simulink model "nxtway_gs_plant"  (Simulink 10.0)
settings: Solver=ode45  StartTime=0.0  StopTime=10.0  MaxStep=TS  RelTol=1e-3  EnableMultiTasking=on
PreLoadFcn:
  | param_nxtway_gs
undefined symbols (not defined in the file): A1, A2, B1, B2, C1, C2, D1, D2, X1IV, X2IV
settings Model: Creator=y_yama  LastModifiedBy=bhisma
settings DataIOCC: LimitDataPoints=on  SignalLoggingSaveFormat=ModelDataLogs  SaveOutput=off  SignalLogging=off  SaveTime=off
settings OptimizationCC: DefaultParameterBehavior=Inlined  InlineInvariantSignals=on  ExpressionDepthLimit=2147483647  InitFltsAndDblsToZero=on  LifeSpan=1
settings DebuggingCC: SolverPrmCheckMsg=warning  FcnCallInpInsideContextMsg=warning  StateNameClashWarn=warning
settings HardwareCC: ProdLargestAtomicInteger=Long  ProdLargestAtomicFloat=Float  ProdIntDivRoundTo=Zero  ProdEndianess=LittleEndian  ProdHWDeviceType=ARM Compatible->ARM 7
settings SFSimCC: SimUseLocalCustomCode=on  CustomCodeUndefinedFunction=FilterOut
settings RTWCC: RTWUseLocalCustomCode=on

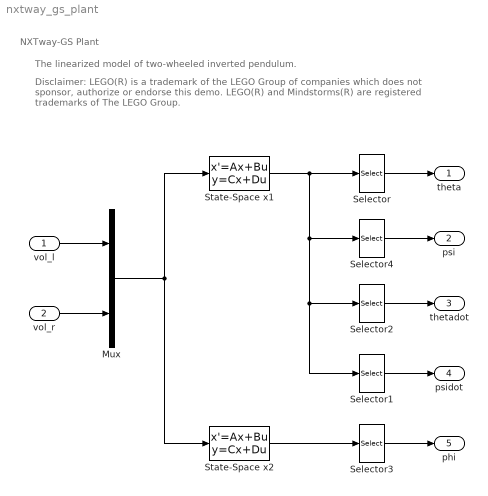
== system nxtway_gs_plant ==
  note: NXTway-GS Plant
  note: The linearized model of two-wheeled inverted pendulum.
  note: Disclaimer:
      | LEGO(R) is a trademark of the LEGO Group of companies which does not sponsor,
      | authorize or endorse this demo.
      | LEGO(R) and Mindstorms(R) are registered trademarks of The LEGO Group.
  vol_l : Inport  OutDataTypeStr=double
  vol_r : Inport  Port=2  OutDataTypeStr=double
  Mux : Mux  Inputs=2
  Selector : Selector  InputPortWidth=4  IndexOptions=Index vector (dialog)  Indices=1  OutputSizes=1
  Selector1 : Selector  InputPortWidth=4  IndexOptions=Index vector (dialog)  Indices=4  OutputSizes=1
  Selector2 : Selector  InputPortWidth=4  IndexOptions=Index vector (dialog)  Indices=3  OutputSizes=1
  Selector3 : Selector  InputPortWidth=2  IndexOptions=Index vector (dialog)  Indices=1  OutputSizes=1
  Selector4 : Selector  InputPortWidth=4  IndexOptions=Index vector (dialog)  Indices=2  OutputSizes=1
  State-Space x1 : StateSpace  A=A1  B=B1  C=C1  D=D1  InitialCondition=X1IV
  State-Space x2 : StateSpace  A=A2  B=B2  C=C2  D=D2  InitialCondition=X2IV
  theta : Outport
  psi : Outport  Port=2
  thetadot : Outport  Port=3
  psidot : Outport  Port=4
  phi : Outport  Port=5
  wires:
  vol_l/1 -> Mux/1
  vol_r/1 -> Mux/2
  Mux/1 -> State-Space x1/1, State-Space x2/1
  State-Space x1/1 -> Selector/1, Selector2/1, Selector1/1, Selector4/1
  State-Space x2/1 -> Selector3/1
  Selector/1 -> theta/1
  Selector3/1 -> phi/1
  Selector2/1 -> thetadot/1
  Selector1/1 -> psidot/1
  Selector4/1 -> psi/1
